simulink model "a2024_V2X_6V_Simulink_model"  (R2023b)
settings: Solver=VariableStepAuto  StartTime=0.0  StopTime=30  MaxStep=1e-2  RelTol=1e-3  AbsTol=1e-3
values from neighbouring files (symbols this model uses):
  b = 1.6    [a2024_v2x_matlab_6veh.m]
  mEgo = 1500    [a2024_v2x_matlab_6veh.m]
  Mode = 1    [a2024_v2x_matlab_6veh.m]    (also in v2x_matlab.m; v2x_matlabV2.m; v2x_matlab_6veh.m; v2x_matlab_R.m)
  pilot = (randi(s,[0 1],pilotsPerSym,1)-0.5)*2    [v2x_matlab.m]
  RxPowerV1 = zeros(sizeEgoWP+2, sizeV1WP+2)    [a2024_v2x_matlab_6veh.m]
  RxPowerV2 = zeros(sizeEgoWP+2, sizeV2WP+2)    [a2024_v2x_matlab_6veh.m]
  RxPowerV3 = zeros(sizeEgoWP+2, sizeV3WP+2)    [a2024_v2x_matlab_6veh.m]
  RxPowerV4 = zeros(sizeEgoWP+2, sizeV4WP+2)    [a2024_v2x_matlab_6veh.m]
  RxPowerV5 = zeros(sizeEgoWP+2, sizeV5WP+2)    [a2024_v2x_matlab_6veh.m]
  RxPowerV6 = zeros(sizeEgoWP+2, sizeV6WP+2)    [a2024_v2x_matlab_6veh.m]
  sampleTime = 0.1    [a2024_v2x_matlab_6veh.m]    (also in v2x_matlab.m; v2x_matlabV2.m; v2x_matlab_6veh.m; v2x_matlab_R.m)
  t_gap = 1.4    [a2024_v2x_matlab_6veh.m]
  waypoints = [egoWP(:,2) egoWP(:,1), zeroforwp]    [a2024_v2x_matlab_6veh.m]    (also in misc.m = data.data.ActorSpecifications(1,1).Waypoints(:,[1,2]); v2x_matlab.m = data.data.ActorSpecifications(1,1).Waypoints(:,[1,2]); v2x_matlabV2.m = [5 -1.6 0; v2x_matlab_R.m = [5 -1.6 0)
  ZeroActors = struct(     'ActorID',0,     'Position', [1000 1000 1000],      'Velocity', [0 0 0],      'Roll', 0,      'Pitch', 0,      'Yaw', 0,      'AngularVelocity', [0 0 0])    [v2x_matlabV2.m]    (also in v2x_matlab_R.m)
undefined symbols (not defined in the file or in its folder): driving, PredictionHorizon, Ts
libraries: commofdm x50, commcnvcod2 x39, simulink x34, commdigbbndam3 x31, commblkintrlv2 x26, commdigbbndpm3 x14, simulink_extras x12, drivingscenarioandsensors x3, mpcadaslib x2, commchan3 x1, vehdynlibdriver x1, commrandsrc3 x1
(part 6 of 6)

== matlab function a2024_V2X_6V_Simulink_model/Calculate PDR/PDR V2/MATLAB Function1 ==
  data: u input; y output; Vehicle_ID input
function y = fcn(u, Vehicle_ID)

y = u(:,Vehicle_ID);

== matlab function a2024_V2X_6V_Simulink_model/Calculate PDR/PDR V2/MATLAB Function2 ==
  settings: sampleTime=sampleTime
  data: Vehicle_ID input; u input; y output
function y = fcn(Vehicle_ID, u)

if isempty(u(:,Vehicle_ID)) 
    y = zeros(1,16);
else
    y = u(:,Vehicle_ID);
end

end

== matlab function a2024_V2X_6V_Simulink_model/Subsystem/MATLAB Function1 ==
  settings: sampleTime=inherited
  data: busActors3Test1 input; Actor output size=18; VehicleID input; VehicleData output Bus: Actors; EgoData input Bus: Actors; counter output; rxPower output; RxPower input
  events: trigger input RISING_EDGE_EVENT
function [Actor, VehicleData, counter, rxPower]  = convBus2IntVector(busActors3Test1, VehicleID, EgoData, RxPower)

% Data extracted from actorss bus

%ActorId = BusActors1Actors.Actors(ActorID).ActorID(1:1);
numActors = int16(busActors3Test1.NumActors);
%time = busActors3Test1.Time;
time = int16(busActors3Test1.Time);

ActorID = VehicleID;

posX = busActors3Test1.Actors(ActorID).Position(1:1);
posY = busActors3Test1.Actors(ActorID).Position(2:2);
posZ = busActors3Test1.Actors(ActorID).Position(3:3);
vPos = [posX posY posZ];

vX = busActors3Test1.Actors(ActorID).Velocity(1:1);
vY = busActors3Test1.Actors(ActorID).Velocity(2:2);
vZ = busActors3Test1.Actors(ActorID).Velocity(3:3);

roll = busActors3Test1.Actors(ActorID).Roll(1:1);
pitch = busActors3Test1.Actors(ActorID).Pitch(1:1);
yaw = busActors3Test1.Actors(ActorID).Yaw(1:1);


angularVelocityX = busActors3Test1.Actors(ActorID).AngularVelocity(1:1);
angularVelocityY = busActors3Test1.Actors(ActorID).AngularVelocity(2:2);
angularVelocityZ = busActors3Test1.Actors(ActorID).AngularVelocity(3:3);

VehicleData = busActors3Test1.Actors(VehicleID);


%% Converting the data

ActorID = int16(ActorID)*10;

posMultip = 10;
posX = int16(round(posMultip*posX));
posY = int16(round(posMultip*posY));
posZ = int16(round(posMultip*posZ));

velMultip = 50;
vX = int16(round(velMultip * vX));
vY = int16(round(velMultip * vY));
vZ = int16(round(velMultip * vZ));

rpyMultip = 50;
roll = int16(round(rpyMultip * roll));
pitch = int16(round(rpyMultip * pitch));
yaw = int16(round(rpyMultip * yaw));

angvelMultip = 50;
angularVelocityX = int16(round(angvelMultip * angularVelocityX));
angularVelocityY = int16(round(angvelMultip * angularVelocityY));
angularVelocityZ = int16(round(angvelMultip * angularVelocityZ));

minusones = ones(3,1);
% Output vector
%zerosVector = zeros(9,1);

intVector = [numActors; time; ActorID; posX; posY; posZ; vX; vY; vZ; roll; pitch; yaw; angularVelocityX; angularVelocityY; angularVelocityZ; minusones];

Actor = intVector;

%% Pathloss (freespace)

% EgoPos = [EgoData.Position(2) EgoData.Position(1) EgoData.Position(3)];
EgoPos = EgoData.Position;
dist = norm(vPos - EgoPos);

fc = 5.9e9;  % Carrier frequency
lambda = (physconst('LightSpeed'))/fc;

PL = fspl(dist, lambda);

Pt_dBm = 33;    % [dBm] Transmission power; maximum permissible transmit power level
sigma = rand(1) + 3.2;  % [3.7 +- 0.5] Variance of the shadowing effect in the wireless communication channel
                        % shadowing follows a log-normal random distribution
X = 2*rand(1)-1;      % random variable following a normal distribution with mean 0 and standard deviation 1
SH = sigma * X;

% h_T = 1;
% h_R = 1;
% dF =  (4*h_T*h_R)/lambda
% lambda1 = 1.61; % Pathloss exponent LOS
% lambda2 = 1.85; % Pathloss exponent NLOS

Pr = Pt_dBm - PL - SH; 

% l1 = 10*lambda1*log(dF)
% l2 = 10*lambda2*log(dist/dF)
% Pr = Prt - l1 - l2 + SH;

P_SEN = -60;

%ZeroActors = int16(zeros(15,1));
% 
counter = 0;
% storedPacket = int16(nan(15,1));
% 
% if Pr > P_SEN
%     Actor = intVector;
%     storedPacket = intVector;
%     counter = 0;
% elseif counter < 10
%     Actor = storedPacket;
%     counter = counter + 1;
% end


%disp(storedPacket)


% persistent prev_value;
% if isempty(prev_value)
%     prev_value = int16(nan(15,1)); % Initialize to a default value
% end
% 
% if Pr > P_SEN
%     Actor = intVector;
%     prev_value = intVector;
%     counter = 0;
% elseif counter < 1
%     Actor = prev_value;
%     counter = counter + 1;
% end


%% SNR
bandwidth = 10e6;
F = 6; % [dB] Noise figure
k = physconst('Boltzmann'); % Boltzmann állandó
T = 300; % [K] Abszolút hőmérséklet

%N0 = 10*log10(bandwidth*k*T/1000)
N0 = -103.8277942;


%N0 = -99;
%SNR = Pr - N0;
egoposition = EgoPos(1,1:2);


distEGO = sqrt(sum((RxPower(3:end, 1:2) - EgoPos(1,1:2)).^2, 2));
distV = sqrt(sum((RxPower(1:2, 3:end)' - vPos(1,1:2)).^2, 2));

[EGOvalue, closestEGO] = min(distEGO);
[Vvalue, closestV] = min(distV);


rxPower = RxPower(closestEGO+2, closestV+2);


%SNR = rxPower - N0;

%% Packet counter
counter = 0;

if (Pr > P_SEN)
    counter = counter + 1;
end

end

== matlab function a2024_V2X_6V_Simulink_model/Calculate PDR/PDR V2/MATLAB Function6 ==
  data: u input; y output Bus: Actors; vehicleID input
function y = fcn(u,vehicleID)

actorsCount = size(u,1);

MinusOneActor = struct(...
    'ActorID',0,...
    'Position', [0 0 0], ...
    'Velocity', [0 0 0], ...
    'Roll', 0, ...
    'Pitch', 0, ...
    'Yaw', 0, ...
    'AngularVelocity', [0 0 0]);

if actorsCount < vehicleID
    y = MinusOneActor;
else
    y = u(:,vehicleID);
end
end

== matlab function a2024_V2X_6V_Simulink_model/Calculate PDR/PDR V3/MATLAB Function ==
  settings: updateMethod=DISCRETE  sampleTime=sampleTime
  data: Tx input; PDR output; Rx input
function PDR = PDR(Tx, Rx)

    
    persistent N S Tx_buffer Rx_buffer

    buffer_size = 20;

    if isempty(N) || isempty(S) || isempty(Tx_buffer) || isempty(Rx_buffer)
        N = 0;
        S = 0;
        Tx_buffer = int16(zeros(buffer_size, length(Tx)));
        Rx_buffer = int16(zeros(buffer_size, length(Rx)));
    end

    Tx_buffer = [Tx_buffer(2:end, :); Tx'];
    Rx_buffer = [Rx_buffer(2:end, :); Rx'];

    if isequal(Tx, Rx) % Check if the entire vectors are the same
        N = N + 1;      % Increment the correct packet count
    end
    S = S + 1;          % Increment the total count
    
    % Calculate the PDR for the last 10 packets
    N_last10 = sum(all(Tx_buffer == Rx_buffer, 2));
    S_last10 = buffer_size;
    R_last10 = (N_last10/S_last10)*100; % Calculate the packet delivery rate [%] for the last 10 packets
    
    R = (N/S)*100;       % Calculate the packet delivery rate [%]
    PDR = [R; N; S; R_last10];
end

== matlab function a2024_V2X_6V_Simulink_model/Calculate PDR/PDR V3/MATLAB Function1 ==
  data: u input; y output; Vehicle_ID input
function y = fcn(u, Vehicle_ID)

y = u(:,Vehicle_ID);

== matlab function a2024_V2X_6V_Simulink_model/Calculate PDR/PDR V3/MATLAB Function2 ==
  settings: sampleTime=sampleTime
  data: Vehicle_ID input; u input; y output
function y = fcn(Vehicle_ID, u)

if isempty(u(:,Vehicle_ID)) 
    y = zeros(1,16);
else
    y = u(:,Vehicle_ID);
end

end

== matlab function a2024_V2X_6V_Simulink_model/Calculate PDR/PDR V3/MATLAB Function6 ==
  data: u input; y output Bus: Actors; vehicleID input
function y = fcn(u,vehicleID)

actorsCount = size(u,1);

MinusOneActor = struct(...
    'ActorID',0,...
    'Position', [0 0 0], ...
    'Velocity', [0 0 0], ...
    'Roll', 0, ...
    'Pitch', 0, ...
    'Yaw', 0, ...
    'AngularVelocity', [0 0 0]);

if actorsCount < vehicleID
    y = MinusOneActor;
else
    y = u(:,vehicleID);
end
end

== matlab function a2024_V2X_6V_Simulink_model/Calculate PDR/PDR V4/MATLAB Function ==
  settings: updateMethod=DISCRETE  sampleTime=sampleTime
  data: Tx input; PDR output; Rx input
function PDR = PDR(Tx, Rx)

    
    persistent N S Tx_buffer Rx_buffer

    buffer_size = 20;

    if isempty(N) || isempty(S) || isempty(Tx_buffer) || isempty(Rx_buffer)
        N = 0;
        S = 0;
        Tx_buffer = int16(zeros(buffer_size, length(Tx)));
        Rx_buffer = int16(zeros(buffer_size, length(Rx)));
    end

    Tx_buffer = [Tx_buffer(2:end, :); Tx'];
    Rx_buffer = [Rx_buffer(2:end, :); Rx'];

    if isequal(Tx, Rx) % Check if the entire vectors are the same
        N = N + 1;      % Increment the correct packet count
    end
    S = S + 1;          % Increment the total count
    
    % Calculate the PDR for the last 10 packets
    N_last10 = sum(all(Tx_buffer == Rx_buffer, 2));
    S_last10 = buffer_size;
    R_last10 = (N_last10/S_last10)*100; % Calculate the packet delivery rate [%] for the last 10 packets
    
    R = (N/S)*100;       % Calculate the packet delivery rate [%]
    PDR = [R; N; S; R_last10];
end

== matlab function a2024_V2X_6V_Simulink_model/Calculate PDR/PDR V4/MATLAB Function1 ==
  data: u input; y output; Vehicle_ID input
function y = fcn(u, Vehicle_ID)

y = u(:,Vehicle_ID);

== matlab function a2024_V2X_6V_Simulink_model/Calculate PDR/PDR V4/MATLAB Function2 ==
  settings: sampleTime=sampleTime
  data: Vehicle_ID input; u input; y output
function y = fcn(Vehicle_ID, u)

if isempty(u(:,Vehicle_ID)) 
    y = zeros(1,16);
else
    y = u(:,Vehicle_ID);
end

end

== matlab function a2024_V2X_6V_Simulink_model/Calculate PDR/PDR V1/MATLAB Function ==
  settings: updateMethod=DISCRETE  sampleTime=sampleTime
  data: Tx input; PDR output; Rx input
function PDR = PDR(Tx, Rx)

    
    persistent N S Tx_buffer Rx_buffer

    buffer_size = 20;

    if isempty(N) || isempty(S) || isempty(Tx_buffer) || isempty(Rx_buffer)
        N = 0;
        S = 0;
        Tx_buffer = int16(zeros(buffer_size, length(Tx)));
        Rx_buffer = int16(zeros(buffer_size, length(Rx)));
    end

    Tx_buffer = [Tx_buffer(2:end, :); Tx'];
    Rx_buffer = [Rx_buffer(2:end, :); Rx'];

    if isequal(Tx, Rx) % Check if the entire vectors are the same
        N = N + 1;      % Increment the correct packet count
    end
    S = S + 1;          % Increment the total count
    
    % Calculate the PDR for the last 10 packets
    N_last10 = sum(all(Tx_buffer == Rx_buffer, 2));
    S_last10 = buffer_size;
    R_last10 = (N_last10/S_last10)*100; % Calculate the packet delivery rate [%] for the last 10 packets
    
    R = (N/S)*100;       % Calculate the packet delivery rate [%]
    PDR = [R; N; S; R_last10];
end

== matlab function a2024_V2X_6V_Simulink_model/Calculate PDR/PDR V1/MATLAB Function2 ==
  settings: sampleTime=sampleTime
  data: Vehicle_ID input; u input; y output
function y = fcn(Vehicle_ID, u)

if isempty(u(:,Vehicle_ID)) 
    y = zeros(1,16);
else
    y = u(:,Vehicle_ID);
end

end

== matlab function a2024_V2X_6V_Simulink_model/Calculate PDR/PDR V1/MATLAB Function6 ==
  data: u input; y output Bus: Actors; vehicleID input
function y = fcn(u,vehicleID)

actorsCount = size(u,1);

MinusOneActor = struct(...
    'ActorID',0,...
    'Position', [0 0 0], ...
    'Velocity', [0 0 0], ...
    'Roll', 0, ...
    'Pitch', 0, ...
    'Yaw', 0, ...
    'AngularVelocity', [0 0 0]);

if actorsCount < vehicleID
    y = MinusOneActor;
else
    y = u(:,vehicleID);
end
end

== matlab function a2024_V2X_6V_Simulink_model/Calculate PDR/PDR V4/MATLAB Function6 ==
  data: u input; y output Bus: Actors; vehicleID input
function y = fcn(u,vehicleID)

actorsCount = size(u,1);

MinusOneActor = struct(...
    'ActorID',0,...
    'Position', [0 0 0], ...
    'Velocity', [0 0 0], ...
    'Roll', 0, ...
    'Pitch', 0, ...
    'Yaw', 0, ...
    'AngularVelocity', [0 0 0]);

if actorsCount < vehicleID
    y = MinusOneActor;
else
    y = u(:,vehicleID);
end
end

== matlab function a2024_V2X_6V_Simulink_model/Calculate PDR/PDR V5/MATLAB Function ==
  settings: updateMethod=DISCRETE  sampleTime=sampleTime
  data: Tx input; PDR output; Rx input
function PDR = PDR(Tx, Rx)

    
    persistent N S Tx_buffer Rx_buffer

    buffer_size = 20;

    if isempty(N) || isempty(S) || isempty(Tx_buffer) || isempty(Rx_buffer)
        N = 0;
        S = 0;
        Tx_buffer = int16(zeros(buffer_size, length(Tx)));
        Rx_buffer = int16(zeros(buffer_size, length(Rx)));
    end

    Tx_buffer = [Tx_buffer(2:end, :); Tx'];
    Rx_buffer = [Rx_buffer(2:end, :); Rx'];

    if isequal(Tx, Rx) % Check if the entire vectors are the same
        N = N + 1;      % Increment the correct packet count
    end
    S = S + 1;          % Increment the total count
    
    % Calculate the PDR for the last 10 packets
    N_last10 = sum(all(Tx_buffer == Rx_buffer, 2));
    S_last10 = buffer_size;
    R_last10 = (N_last10/S_last10)*100; % Calculate the packet delivery rate [%] for the last 10 packets
    
    R = (N/S)*100;       % Calculate the packet delivery rate [%]
    PDR = [R; N; S; R_last10];
end

== matlab function a2024_V2X_6V_Simulink_model/Calculate PDR/PDR V5/MATLAB Function1 ==
  data: u input; y output; Vehicle_ID input
function y = fcn(u, Vehicle_ID)

y = u(:,Vehicle_ID);

== matlab function a2024_V2X_6V_Simulink_model/Subsystem7/MATLAB Function2 ==
  settings: sampleTime=sampleTime
  data: input input; Actors output
function Actors = getRealValues(input) 

modulated = input;

NumActors = modulated(1,:);
Time = modulated(2,:);

ActorID = modulated(3,1)/10;

posMultip = 10;  % 10
posX = (modulated(4,:)/posMultip);
posY = (modulated(5,:)/posMultip);
posZ = (modulated(6,:)/posMultip);

velMultip = 50;  % 50
vX = (modulated(7,:)/velMultip);
vY = (modulated(8,:)/velMultip);
vZ = (modulated(9,:)/velMultip);

rpyMultip = 50;  % 50
Roll = (modulated(10,:)/rpyMultip);
Pitch = (modulated(11,:)/rpyMultip);
Yaw = (modulated(12,:)/rpyMultip);

angvelMultip = 50;  % 50
angularVelocityX = (modulated(13,:)/angvelMultip);
angularVelocityY = (modulated(14,:)/angvelMultip);
angularVelocityZ = (modulated(15,:)/angvelMultip);

% Velocity = [vX vY vZ];
% Position = [posX posY posZ];
% AngularVelocity = [angularVelocityX; angularVelocityY; angularVelocityZ];


%Actors = [NumActors; Time; ActorID; Position; Velocity; Roll; Pitch; Yaw; AngularVelocity];
Actors = [NumActors; Time; ActorID; posX; posY; posZ; vX; vY; vZ; Roll; Pitch; Yaw; angularVelocityX; angularVelocityY; angularVelocityZ];


end

== matlab function a2024_V2X_6V_Simulink_model/Subsystem8/MATLAB Function ==
  settings: updateMethod=DISCRETE  sampleTime=sampleTime
  data: SNR input; modulated input; disrupted_Signal output
function disrupted_Signal = PRO_error(SNR, modulated)

disrupted_Signal = awgn(modulated,SNR, -10);

== matlab function a2024_V2X_6V_Simulink_model/Subsystem8/MATLAB Function1 ==
  settings: sampleTime=inherited
  data: busActors3Test1 input; Actor output size=18; VehicleID input; VehicleData output Bus: Actors; EgoData input Bus: Actors; counter output; rxPower output; RxPower input
  events: trigger input RISING_EDGE_EVENT
function [Actor, VehicleData, counter, rxPower]  = convBus2IntVector(busActors3Test1, VehicleID, EgoData, RxPower)

% Data extracted from actorss bus

%ActorId = BusActors1Actors.Actors(ActorID).ActorID(1:1);
numActors = int16(busActors3Test1.NumActors);
%time = busActors3Test1.Time;
time = int16(busActors3Test1.Time);

ActorID = VehicleID;

posX = busActors3Test1.Actors(ActorID).Position(1:1);
posY = busActors3Test1.Actors(ActorID).Position(2:2);
posZ = busActors3Test1.Actors(ActorID).Position(3:3);
vPos = [posX posY posZ];

vX = busActors3Test1.Actors(ActorID).Velocity(1:1);
vY = busActors3Test1.Actors(ActorID).Velocity(2:2);
vZ = busActors3Test1.Actors(ActorID).Velocity(3:3);

roll = busActors3Test1.Actors(ActorID).Roll(1:1);
pitch = busActors3Test1.Actors(ActorID).Pitch(1:1);
yaw = busActors3Test1.Actors(ActorID).Yaw(1:1);


angularVelocityX = busActors3Test1.Actors(ActorID).AngularVelocity(1:1);
angularVelocityY = busActors3Test1.Actors(ActorID).AngularVelocity(2:2);
angularVelocityZ = busActors3Test1.Actors(ActorID).AngularVelocity(3:3);

VehicleData = busActors3Test1.Actors(VehicleID);


%% Converting the data

ActorID = int16(ActorID)*10;

posMultip = 10;
posX = int16(round(posMultip*posX));
posY = int16(round(posMultip*posY));
posZ = int16(round(posMultip*posZ));

velMultip = 50;
vX = int16(round(velMultip * vX));
vY = int16(round(velMultip * vY));
vZ = int16(round(velMultip * vZ));

rpyMultip = 50;
roll = int16(round(rpyMultip * roll));
pitch = int16(round(rpyMultip * pitch));
yaw = int16(round(rpyMultip * yaw));

angvelMultip = 50;
angularVelocityX = int16(round(angvelMultip * angularVelocityX));
angularVelocityY = int16(round(angvelMultip * angularVelocityY));
angularVelocityZ = int16(round(angvelMultip * angularVelocityZ));

minusones = ones(3,1);
% Output vector
%zerosVector = zeros(9,1);

intVector = [numActors; time; ActorID; posX; posY; posZ; vX; vY; vZ; roll; pitch; yaw; angularVelocityX; angularVelocityY; angularVelocityZ; minusones];

Actor = intVector;

%% Pathloss (freespace)

EgoPos = EgoData.Position;
dist = norm(vPos - EgoPos);

fc = 5.9e9;  % Carrier frequency
lambda = (physconst('LightSpeed'))/fc;

PL = fspl(dist, lambda);

Pt_dBm = 33;    % [dBm] Transmission power; maximum permissible transmit power level
sigma = rand(1) + 3.2;  % [3.7 +- 0.5] Variance of the shadowing effect in the wireless communication channel
                        % shadowing follows a log-normal random distribution
X = 2*rand(1)-1;      % random variable following a normal distribution with mean 0 and standard deviation 1
SH = sigma * X;

% h_T = 1;
% h_R = 1;
% dF =  (4*h_T*h_R)/lambda
% lambda1 = 1.61; % Pathloss exponent LOS
% lambda2 = 1.85; % Pathloss exponent NLOS

Pr = Pt_dBm - PL - SH; 

% l1 = 10*lambda1*log(dF)
% l2 = 10*lambda2*log(dist/dF)
% Pr = Prt - l1 - l2 + SH;

P_SEN = -60;

%ZeroActors = int16(zeros(15,1));
% 
counter = 0;
% storedPacket = int16(nan(15,1));
% 
% if Pr > P_SEN
%     Actor = intVector;
%     storedPacket = intVector;
%     counter = 0;
% elseif counter < 10
%     Actor = storedPacket;
%     counter = counter + 1;
% end


%disp(storedPacket)


% persistent prev_value;
% if isempty(prev_value)
%     prev_value = int16(nan(15,1)); % Initialize to a default value
% end
% 
% if Pr > P_SEN
%     Actor = intVector;
%     prev_value = intVector;
%     counter = 0;
% elseif counter < 1
%     Actor = prev_value;
%     counter = counter + 1;
% end


%% SNR
bandwidth = 10e6;
F = 6; % [dB] Noise figure
k = physconst('Boltzmann'); % Boltzmann állandó
T = 300; % [K] Abszolút hőmérséklet

%N0 = 10*log10(bandwidth*k*T/1000)
N0 = -103.8277942;


%N0 = -99;
%SNR = Pr - N0;
egoposition = EgoPos(1,1:2);


distEGO = sqrt(sum((RxPower(3:end, 1:2) - EgoPos(1,1:2)).^2, 2));
distV = sqrt(sum((RxPower(1:2, 3:end)' - vPos(1,1:2)).^2, 2));

[EGOvalue, closestEGO] = min(distEGO);
[Vvalue, closestV] = min(distV);


rxPower = RxPower(closestEGO+2, closestV+2);


%SNR = rxPower - N0;

%% Packet counter
counter = 0;

if (Pr > P_SEN)
    counter = counter + 1;
end

end

== matlab function a2024_V2X_6V_Simulink_model/Subsystem3/MATLAB Function2 ==
  settings: sampleTime=sampleTime
  data: input input; Actors output
function Actors = getRealValues(input) 

modulated = input(1:15);

NumActors = modulated(1,:);
Time = modulated(2,:);

ActorID = ((modulated(3,1))/10);

posMultip = 10;  % 10
posX = (modulated(4,:)/posMultip);
posY = (modulated(5,:)/posMultip);
posZ = (modulated(6,:)/posMultip);

velMultip = 50;  % 50
vX = (modulated(7,:)/velMultip);
vY = (modulated(8,:)/velMultip);
vZ = (modulated(9,:)/velMultip);

rpyMultip = 50;  % 50
Roll = (modulated(10,:)/rpyMultip);
Pitch = (modulated(11,:)/rpyMultip);
Yaw = (modulated(12,:)/rpyMultip);

angvelMultip = 50;  % 50
angularVelocityX = (modulated(13,:)/angvelMultip);
angularVelocityY = (modulated(14,:)/angvelMultip);
angularVelocityZ = (modulated(15,:)/angvelMultip);

% Velocity = [vX vY vZ];
% Position = [posX posY posZ];
% AngularVelocity = [angularVelocityX; angularVelocityY; angularVelocityZ];


%Actors = [NumActors; Time; ActorID; Position; Velocity; Roll; Pitch; Yaw; AngularVelocity];
Actors = [NumActors; Time; ActorID; posX; posY; posZ; vX; vY; vZ; Roll; Pitch; Yaw; angularVelocityX; angularVelocityY; angularVelocityZ];


end

== matlab function a2024_V2X_6V_Simulink_model/Subsystem8/MATLAB Function2 ==
  settings: sampleTime=sampleTime
  data: input input; Actors output
function Actors = getRealValues(input) 

modulated = input;

NumActors = modulated(1,:);
Time = modulated(2,:);

ActorID = modulated(3,1)/10;

posMultip = 10;  % 10
posX = (modulated(4,:)/posMultip);
posY = (modulated(5,:)/posMultip);
posZ = (modulated(6,:)/posMultip);

velMultip = 50;  % 50
vX = (modulated(7,:)/velMultip);
vY = (modulated(8,:)/velMultip);
vZ = (modulated(9,:)/velMultip);

rpyMultip = 50;  % 50
Roll = (modulated(10,:)/rpyMultip);
Pitch = (modulated(11,:)/rpyMultip);
Yaw = (modulated(12,:)/rpyMultip);

angvelMultip = 50;  % 50
angularVelocityX = (modulated(13,:)/angvelMultip);
angularVelocityY = (modulated(14,:)/angvelMultip);
angularVelocityZ = (modulated(15,:)/angvelMultip);

% Velocity = [vX vY vZ];
% Position = [posX posY posZ];
% AngularVelocity = [angularVelocityX; angularVelocityY; angularVelocityZ];


%Actors = [NumActors; Time; ActorID; Position; Velocity; Roll; Pitch; Yaw; AngularVelocity];
Actors = [NumActors; Time; ActorID; posX; posY; posZ; vX; vY; vZ; Roll; Pitch; Yaw; angularVelocityX; angularVelocityY; angularVelocityZ];


end

== matlab function a2024_V2X_6V_Simulink_model/Calculate PDR/PDR V5/MATLAB Function2 ==
  settings: sampleTime=sampleTime
  data: Vehicle_ID input; u input; y output
function y = fcn(Vehicle_ID, u)

if isempty(u(:,Vehicle_ID)) 
    y = zeros(1,16);
else
    y = u(:,Vehicle_ID);
end

end

== matlab function a2024_V2X_6V_Simulink_model/Calculate PDR/PDR V5/MATLAB Function6 ==
  data: u input; y output Bus: Actors; vehicleID input
function y = fcn(u,vehicleID)

actorsCount = size(u,1);

MinusOneActor = struct(...
    'ActorID',0,...
    'Position', [0 0 0], ...
    'Velocity', [0 0 0], ...
    'Roll', 0, ...
    'Pitch', 0, ...
    'Yaw', 0, ...
    'AngularVelocity', [0 0 0]);

if actorsCount < vehicleID
    y = MinusOneActor;
else
    y = u(:,vehicleID);
end
end

== matlab function a2024_V2X_6V_Simulink_model/Subsystem9/MATLAB Function2 ==
  settings: sampleTime=sampleTime
  data: input input; Actors output
function Actors = getRealValues(input) 

modulated = input(1:15);

NumActors = modulated(1,:);
Time = modulated(2,:);

ActorID = ((modulated(3,1))/10);

posMultip = 10;  % 10
posX = (modulated(4,:)/posMultip);
posY = (modulated(5,:)/posMultip);
posZ = (modulated(6,:)/posMultip);

velMultip = 50;  % 50
vX = (modulated(7,:)/velMultip);
vY = (modulated(8,:)/velMultip);
vZ = (modulated(9,:)/velMultip);

rpyMultip = 50;  % 50
Roll = (modulated(10,:)/rpyMultip);
Pitch = (modulated(11,:)/rpyMultip);
Yaw = (modulated(12,:)/rpyMultip);

angvelMultip = 50;  % 50
angularVelocityX = (modulated(13,:)/angvelMultip);
angularVelocityY = (modulated(14,:)/angvelMultip);
angularVelocityZ = (modulated(15,:)/angvelMultip);

% Velocity = [vX vY vZ];
% Position = [posX posY posZ];
% AngularVelocity = [angularVelocityX; angularVelocityY; angularVelocityZ];


%Actors = [NumActors; Time; ActorID; Position; Velocity; Roll; Pitch; Yaw; AngularVelocity];
Actors = [NumActors; Time; ActorID; posX; posY; posZ; vX; vY; vZ; Roll; Pitch; Yaw; angularVelocityX; angularVelocityY; angularVelocityZ];


end

== matlab function a2024_V2X_6V_Simulink_model/Calculate PDR/PDR V6/MATLAB Function ==
  settings: updateMethod=DISCRETE  sampleTime=sampleTime
  data: Tx input; PDR output; Rx input
function PDR = PDR(Tx, Rx)

    
    persistent N S Tx_buffer Rx_buffer

    buffer_size = 20;

    if isempty(N) || isempty(S) || isempty(Tx_buffer) || isempty(Rx_buffer)
        N = 0;
        S = 0;
        Tx_buffer = int16(zeros(buffer_size, length(Tx)));
        Rx_buffer = int16(zeros(buffer_size, length(Rx)));
    end

    Tx_buffer = [Tx_buffer(2:end, :); Tx'];
    Rx_buffer = [Rx_buffer(2:end, :); Rx'];

    if isequal(Tx, Rx) % Check if the entire vectors are the same
        N = N + 1;      % Increment the correct packet count
    end
    S = S + 1;          % Increment the total count
    
    % Calculate the PDR for the last 10 packets
    N_last10 = sum(all(Tx_buffer == Rx_buffer, 2));
    S_last10 = buffer_size;
    R_last10 = (N_last10/S_last10)*100; % Calculate the packet delivery rate [%] for the last 10 packets
    
    R = (N/S)*100;       % Calculate the packet delivery rate [%]
    PDR = [R; N; S; R_last10];
end

== matlab function a2024_V2X_6V_Simulink_model/Calculate PDR/PDR V6/MATLAB Function1 ==
  data: u input; y output; Vehicle_ID input
function y = fcn(u, Vehicle_ID)

y = u(:,Vehicle_ID);

== matlab function a2024_V2X_6V_Simulink_model/Calculate PDR/PDR V6/MATLAB Function2 ==
  settings: sampleTime=sampleTime
  data: Vehicle_ID input; u input; y output
function y = fcn(Vehicle_ID, u)

if isempty(u(:,Vehicle_ID)) 
    y = zeros(1,16);
else
    y = u(:,Vehicle_ID);
end

end

== matlab function a2024_V2X_6V_Simulink_model/Calculate PDR/PDR V6/MATLAB Function6 ==
  data: u input; y output Bus: Actors; vehicleID input
function y = fcn(u,vehicleID)

actorsCount = size(u,1);

MinusOneActor = struct(...
    'ActorID',0,...
    'Position', [0 0 0], ...
    'Velocity', [0 0 0], ...
    'Roll', 0, ...
    'Pitch', 0, ...
    'Yaw', 0, ...
    'AngularVelocity', [0 0 0]);

if actorsCount < vehicleID
    y = MinusOneActor;
else
    y = u(:,vehicleID);
end
end

== matlab function a2024_V2X_6V_Simulink_model/Subsystem10/MATLAB Function2 ==
  settings: sampleTime=sampleTime
  data: input input; Actors output
function Actors = getRealValues(input) 

modulated = input(1:15);

NumActors = modulated(1,:);
Time = modulated(2,:);

ActorID = ((modulated(3,1))/10);

posMultip = 10;  % 10
posX = (modulated(4,:)/posMultip);
posY = (modulated(5,:)/posMultip);
posZ = (modulated(6,:)/posMultip);

velMultip = 50;  % 50
vX = (modulated(7,:)/velMultip);
vY = (modulated(8,:)/velMultip);
vZ = (modulated(9,:)/velMultip);

rpyMultip = 50;  % 50
Roll = (modulated(10,:)/rpyMultip);
Pitch = (modulated(11,:)/rpyMultip);
Yaw = (modulated(12,:)/rpyMultip);

angvelMultip = 50;  % 50
angularVelocityX = (modulated(13,:)/angvelMultip);
angularVelocityY = (modulated(14,:)/angvelMultip);
angularVelocityZ = (modulated(15,:)/angvelMultip);

% Velocity = [vX vY vZ];
% Position = [posX posY posZ];
% AngularVelocity = [angularVelocityX; angularVelocityY; angularVelocityZ];


%Actors = [NumActors; Time; ActorID; Position; Velocity; Roll; Pitch; Yaw; AngularVelocity];
Actors = [NumActors; Time; ActorID; posX; posY; posZ; vX; vY; vZ; Roll; Pitch; Yaw; angularVelocityX; angularVelocityY; angularVelocityZ];


end

== matlab function a2024_V2X_6V_Simulink_model/Subsystem4/MATLAB Function ==
  settings: updateMethod=DISCRETE  sampleTime=sampleTime
  data: SNR input; modulated input; disrupted_Signal output
function disrupted_Signal = PRO_error(SNR, modulated)

disrupted_Signal = awgn(modulated,SNR, -10);

== matlab function a2024_V2X_6V_Simulink_model/Subsystem11/MATLAB Function2 ==
  settings: sampleTime=sampleTime
  data: input input; Actors output
function Actors = getRealValues(input) 

modulated = input(1:15);

NumActors = modulated(1,:);
Time = modulated(2,:);

ActorID = ((modulated(3,1))/10);

posMultip = 10;  % 10
posX = (modulated(4,:)/posMultip);
posY = (modulated(5,:)/posMultip);
posZ = (modulated(6,:)/posMultip);

velMultip = 50;  % 50
vX = (modulated(7,:)/velMultip);
vY = (modulated(8,:)/velMultip);
vZ = (modulated(9,:)/velMultip);

rpyMultip = 50;  % 50
Roll = (modulated(10,:)/rpyMultip);
Pitch = (modulated(11,:)/rpyMultip);
Yaw = (modulated(12,:)/rpyMultip);

angvelMultip = 50;  % 50
angularVelocityX = (modulated(13,:)/angvelMultip);
angularVelocityY = (modulated(14,:)/angvelMultip);
angularVelocityZ = (modulated(15,:)/angvelMultip);

% Velocity = [vX vY vZ];
% Position = [posX posY posZ];
% AngularVelocity = [angularVelocityX; angularVelocityY; angularVelocityZ];


%Actors = [NumActors; Time; ActorID; Position; Velocity; Roll; Pitch; Yaw; AngularVelocity];
Actors = [NumActors; Time; ActorID; posX; posY; posZ; vX; vY; vZ; Roll; Pitch; Yaw; angularVelocityX; angularVelocityY; angularVelocityZ];


end

== matlab function a2024_V2X_6V_Simulink_model/Subsystem12/MATLAB Function2 ==
  settings: sampleTime=sampleTime
  data: input input; Actors output
function Actors = getRealValues(input) 

modulated = input(1:15);

NumActors = modulated(1,:);
Time = modulated(2,:);

ActorID = ((modulated(3,1))/10);

posMultip = 10;  % 10
posX = (modulated(4,:)/posMultip);
posY = (modulated(5,:)/posMultip);
posZ = (modulated(6,:)/posMultip);

velMultip = 50;  % 50
vX = (modulated(7,:)/velMultip);
vY = (modulated(8,:)/velMultip);
vZ = (modulated(9,:)/velMultip);

rpyMultip = 50;  % 50
Roll = (modulated(10,:)/rpyMultip);
Pitch = (modulated(11,:)/rpyMultip);
Yaw = (modulated(12,:)/rpyMultip);

angvelMultip = 50;  % 50
angularVelocityX = (modulated(13,:)/angvelMultip);
angularVelocityY = (modulated(14,:)/angvelMultip);
angularVelocityZ = (modulated(15,:)/angvelMultip);

% Velocity = [vX vY vZ];
% Position = [posX posY posZ];
% AngularVelocity = [angularVelocityX; angularVelocityY; angularVelocityZ];


%Actors = [NumActors; Time; ActorID; Position; Velocity; Roll; Pitch; Yaw; AngularVelocity];
Actors = [NumActors; Time; ActorID; posX; posY; posZ; vX; vY; vZ; Roll; Pitch; Yaw; angularVelocityX; angularVelocityY; angularVelocityZ];


end

== matlab function a2024_V2X_6V_Simulink_model/Subsystem13/MATLAB Function2 ==
  settings: sampleTime=sampleTime
  data: input input; Actors output
function Actors = getRealValues(input) 

modulated = input(1:15);

NumActors = modulated(1,:);
Time = modulated(2,:);

ActorID = ((modulated(3,1))/10);

posMultip = 10;  % 10
posX = (modulated(4,:)/posMultip);
posY = (modulated(5,:)/posMultip);
posZ = (modulated(6,:)/posMultip);

velMultip = 50;  % 50
vX = (modulated(7,:)/velMultip);
vY = (modulated(8,:)/velMultip);
vZ = (modulated(9,:)/velMultip);

rpyMultip = 50;  % 50
Roll = (modulated(10,:)/rpyMultip);
Pitch = (modulated(11,:)/rpyMultip);
Yaw = (modulated(12,:)/rpyMultip);

angvelMultip = 50;  % 50
angularVelocityX = (modulated(13,:)/angvelMultip);
angularVelocityY = (modulated(14,:)/angvelMultip);
angularVelocityZ = (modulated(15,:)/angvelMultip);

% Velocity = [vX vY vZ];
% Position = [posX posY posZ];
% AngularVelocity = [angularVelocityX; angularVelocityY; angularVelocityZ];


%Actors = [NumActors; Time; ActorID; Position; Velocity; Roll; Pitch; Yaw; AngularVelocity];
Actors = [NumActors; Time; ActorID; posX; posY; posZ; vX; vY; vZ; Roll; Pitch; Yaw; angularVelocityX; angularVelocityY; angularVelocityZ];


end

== matlab function a2024_V2X_6V_Simulink_model/Subsystem14/MATLAB Function2 ==
  settings: sampleTime=sampleTime
  data: input input; Actors output
function Actors = getRealValues(input) 

modulated = input(1:15);

NumActors = modulated(1,:);
Time = modulated(2,:);

ActorID = ((modulated(3,1))/10);

posMultip = 10;  % 10
posX = (modulated(4,:)/posMultip);
posY = (modulated(5,:)/posMultip);
posZ = (modulated(6,:)/posMultip);

velMultip = 50;  % 50
vX = (modulated(7,:)/velMultip);
vY = (modulated(8,:)/velMultip);
vZ = (modulated(9,:)/velMultip);

rpyMultip = 50;  % 50
Roll = (modulated(10,:)/rpyMultip);
Pitch = (modulated(11,:)/rpyMultip);
Yaw = (modulated(12,:)/rpyMultip);

angvelMultip = 50;  % 50
angularVelocityX = (modulated(13,:)/angvelMultip);
angularVelocityY = (modulated(14,:)/angvelMultip);
angularVelocityZ = (modulated(15,:)/angvelMultip);

% Velocity = [vX vY vZ];
% Position = [posX posY posZ];
% AngularVelocity = [angularVelocityX; angularVelocityY; angularVelocityZ];


%Actors = [NumActors; Time; ActorID; Position; Velocity; Roll; Pitch; Yaw; AngularVelocity];
Actors = [NumActors; Time; ActorID; posX; posY; posZ; vX; vY; vZ; Roll; Pitch; Yaw; angularVelocityX; angularVelocityY; angularVelocityZ];


end

== matlab function a2024_V2X_6V_Simulink_model/MATLAB Function ==
  data: V1Actor input; relDist output; EgoActor input; relVel output; EgoPos output
function [relDist, relVel, EgoPos] = fcn(V1Actor, EgoActor)


EgoPos = double(EgoActor.Position);
EgoVel = double(EgoActor.Velocity);

V1Pos = double(V1Actor(4:6,1))';
V1Vel = double(V1Actor(7:9,1))';

if isequal(V1Pos, zeros(1,3))
    V1Pos = [170 3 0];
    V1Vel = [0, -7, 0];
end


%EgoPosNorm = norm(EgoPos);
%V1PosNorm = norm(V1Pos);

%possquared = (EgoPos(1) - V1Pos(1))^2 + (EgoPos(2) - V1Pos(2))^2;

%EgoVelNorm = norm(EgoVel);
%V1VelNorm = norm(V1Vel);

%velsquared = (EgoVel(1) - V1Vel(1))^2 + (EgoVel(2) - V1Vel(2))^2;

%relDist = sqrt(possquared);
relDist = V1Pos - EgoPos;
%relVel = sqrt(velsquared)
relVel = V1Vel - EgoVel;

% relDist = sqrt((((EgoPos(1) - V1Pos(1)).^2)+((EgoPos(2) - V1Pos(2))).^2), 2);
% relVel = sqrt((((EgoVel(1) - V1Vel(1)).^2)+((EgoVel(2) - V1Vel(2))).^2), 2);

% relDist = norm(V1Pos - EgoPos);
% relVel = norm(V1Vel - EgoVel);

== matlab function a2024_V2X_6V_Simulink_model/Vehicle 3/MATLAB Function2 ==
  data: busActors3Test1 input; intVector output int16 size=15; VehicleID input
  events: trigger input RISING_EDGE_EVENT
function intVector = convBus2IntVector(busActors3Test1, VehicleID)

% Data extracted from actorss bus

%ActorId = BusActors1Actors.Actors(ActorID).ActorID(1:1);
numActors = busActors3Test1.NumActors;
time = busActors3Test1.Time;

ActorID = VehicleID;

posX = busActors3Test1.Actors(ActorID).Position(1:1);
posY = busActors3Test1.Actors(ActorID).Position(2:2);
posZ = busActors3Test1.Actors(ActorID).Position(3:3);

vX = busActors3Test1.Actors(ActorID).Velocity(1:1);
vY = busActors3Test1.Actors(ActorID).Velocity(2:2);
vZ = busActors3Test1.Actors(ActorID).Velocity(3:3);

roll = busActors3Test1.Actors(ActorID).Roll(1:1);
pitch = busActors3Test1.Actors(ActorID).Pitch(1:1);
yaw = busActors3Test1.Actors(ActorID).Yaw(1:1);


angularVelocityX = busActors3Test1.Actors(ActorID).AngularVelocity(1:1);
angularVelocityY = busActors3Test1.Actors(ActorID).AngularVelocity(2:2);
angularVelocityZ = busActors3Test1.Actors(ActorID).AngularVelocity(3:3);


% Converting the data

ActorID = int16(ActorID);

posMultip = 10;
posX = int16(round(posMultip*posX));
posY = int16(round(posMultip*posY));
posZ = int16(round(posMultip*posZ));

velMultip = 50;
vX = int16(round(velMultip * vX));
vY = int16(round(velMultip * vY));
vZ = int16(round(velMultip * vZ));

rpyMultip = 50;
roll = int16(round(rpyMultip * roll));
pitch = int16(round(rpyMultip * pitch));
yaw = int16(round(rpyMultip * yaw));

angvelMultip = 50;
angularVelocityX = int16(round(angvelMultip * angularVelocityX));
angularVelocityY = int16(round(angvelMultip * angularVelocityY));
angularVelocityZ = int16(round(angvelMultip * angularVelocityZ));


% Output vector
%zerosVector = zeros(9,1);

intVector = [numActors; time; ActorID; posX; posY; posZ; vX; vY; vZ; roll; pitch; yaw; angularVelocityX; angularVelocityY; angularVelocityZ];
end

== matlab function a2024_V2X_6V_Simulink_model/Subsystem1/MATLAB Function1 ==
  data: busActors3Test1 input; Actor output int16 size=15; VehicleID input; VehicleData output Bus: Actors; EgoData input Bus: Actors; counter output
  events: trigger input RISING_EDGE_EVENT
function [Actor, VehicleData, counter]  = convBus2IntVector(busActors3Test1, VehicleID, EgoData)

% Data extracted from actorss bus

%ActorId = BusActors1Actors.Actors(ActorID).ActorID(1:1);
numActors = busActors3Test1.NumActors;
%time = busActors3Test1.Time;
time = busActors3Test1.Time;

ActorID = VehicleID;

posX = busActors3Test1.Actors(ActorID).Position(1:1);
posY = busActors3Test1.Actors(ActorID).Position(2:2);
posZ = busActors3Test1.Actors(ActorID).Position(3:3);
vPos = [posX posY posZ];

vX = busActors3Test1.Actors(ActorID).Velocity(1:1);
vY = busActors3Test1.Actors(ActorID).Velocity(2:2);
vZ = busActors3Test1.Actors(ActorID).Velocity(3:3);

roll = busActors3Test1.Actors(ActorID).Roll(1:1);
pitch = busActors3Test1.Actors(ActorID).Pitch(1:1);
yaw = busActors3Test1.Actors(ActorID).Yaw(1:1);


angularVelocityX = busActors3Test1.Actors(ActorID).AngularVelocity(1:1);
angularVelocityY = busActors3Test1.Actors(ActorID).AngularVelocity(2:2);
angularVelocityZ = busActors3Test1.Actors(ActorID).AngularVelocity(3:3);

VehicleData = busActors3Test1.Actors(ActorID);


%% Converting the data

ActorID = int16(ActorID);

posMultip = 10;
posX = int16(round(posMultip*posX));
posY = int16(round(posMultip*posY));
posZ = int16(round(posMultip*posZ));

velMultip = 50;
vX = int16(round(velMultip * vX));
vY = int16(round(velMultip * vY));
vZ = int16(round(velMultip * vZ));

rpyMultip = 50;
roll = int16(round(rpyMultip * roll));
pitch = int16(round(rpyMultip * pitch));
yaw = int16(round(rpyMultip * yaw));

angvelMultip = 50;
angularVelocityX = int16(round(angvelMultip * angularVelocityX));
angularVelocityY = int16(round(angvelMultip * angularVelocityY));
angularVelocityZ = int16(round(angvelMultip * angularVelocityZ));


% Output vector
%zerosVector = zeros(9,1);

intVector = [numActors; time; ActorID; posX; posY; posZ; vX; vY; vZ; roll; pitch; yaw; angularVelocityX; angularVelocityY; angularVelocityZ];



%% Pathloss (freespace)

EgoPos = EgoData.Position;
dist = norm(vPos - EgoPos);

fc = 5.9*10^9;  % Carrier frequency
lambda = physconst('LightSpeed')/fc;

PL = fspl(dist, lambda);

Pt_dBm = 33;    % [dBm] Transmission power; maximum permissible transmit power level
sigma = rand(1) + 3.2;  % [3.7 +- 0.5] Variance of the shadowing effect in the wireless communication channel
                        % shadowing follows a log-normal random distribution
X = randn(1);       % random variable following a normal distribution with mean 0 and standard deviation 1
SH = sigma * X;

Pr = Pt_dBm - PL - SH;

P_SEN = -60;

ZeroActors = int16(zeros(15,1));

persistent prev_value;
if isempty(prev_value)
    prev_value = ZeroActors; % Initialize to a default value
end

if Pr > P_SEN
    Actor = intVector;
    prev_value = intVector;
else
    Actor = prev_value;
end


%% Packet counter
counter = 0;

if (Pr > P_SEN)
    counter = counter + 1;
end


end

== matlab function a2024_V2X_6V_Simulink_model/MATLAB Function2 ==
  data: Ego input; EgoActor output; V1 input; V1Actor output
function [EgoActor, V1Actor] = ENU_to_NED(Ego, V1)

T = [cos(nu) -sin(nu) 0 a;
    cos(alpha)*sin(nu) cos(alpha)*cos(nu) -sin(alpha) -d*sin(alpha);
    sin(alpha)*sin(nu) sin(alpha)*cos(nu) cos(alpha) d*cos(alpha);
    0 0 0 1];

== matlab function a2024_V2X_6V_Simulink_model/Subsystem4/MATLAB Function1 ==
  settings: sampleTime=inherited
  data: busActors3Test1 input; Actor output size=18; VehicleID input; VehicleData output Bus: Actors; EgoData input Bus: Actors; counter output; rxPower output; RxPower input
  events: trigger input RISING_EDGE_EVENT
function [Actor, VehicleData, counter, rxPower]  = convBus2IntVector(busActors3Test1, VehicleID, EgoData, RxPower)

% Data extracted from actorss bus

%ActorId = BusActors1Actors.Actors(ActorID).ActorID(1:1);
numActors = int16(busActors3Test1.NumActors);
%time = busActors3Test1.Time;
time = int16(busActors3Test1.Time);

ActorID = VehicleID;

posX = busActors3Test1.Actors(ActorID).Position(1:1);
posY = busActors3Test1.Actors(ActorID).Position(2:2);
posZ = busActors3Test1.Actors(ActorID).Position(3:3);
vPos = [posX posY posZ];

vX = busActors3Test1.Actors(ActorID).Velocity(1:1);
vY = busActors3Test1.Actors(ActorID).Velocity(2:2);
vZ = busActors3Test1.Actors(ActorID).Velocity(3:3);

roll = busActors3Test1.Actors(ActorID).Roll(1:1);
pitch = busActors3Test1.Actors(ActorID).Pitch(1:1);
yaw = busActors3Test1.Actors(ActorID).Yaw(1:1);


angularVelocityX = busActors3Test1.Actors(ActorID).AngularVelocity(1:1);
angularVelocityY = busActors3Test1.Actors(ActorID).AngularVelocity(2:2);
angularVelocityZ = busActors3Test1.Actors(ActorID).AngularVelocity(3:3);

VehicleData = busActors3Test1.Actors(VehicleID);


%% Converting the data

ActorID = int16(ActorID)*10;

posMultip = 10;
posX = int16(round(posMultip*posX));
posY = int16(round(posMultip*posY));
posZ = int16(round(posMultip*posZ));

velMultip = 50;
vX = int16(round(velMultip * vX));
vY = int16(round(velMultip * vY));
vZ = int16(round(velMultip * vZ));

rpyMultip = 50;
roll = int16(round(rpyMultip * roll));
pitch = int16(round(rpyMultip * pitch));
yaw = int16(round(rpyMultip * yaw));

angvelMultip = 50;
angularVelocityX = int16(round(angvelMultip * angularVelocityX));
angularVelocityY = int16(round(angvelMultip * angularVelocityY));
angularVelocityZ = int16(round(angvelMultip * angularVelocityZ));

minusones = ones(3,1);
% Output vector
%zerosVector = zeros(9,1);

intVector = [numActors; time; ActorID; posX; posY; posZ; vX; vY; vZ; roll; pitch; yaw; angularVelocityX; angularVelocityY; angularVelocityZ; minusones];

Actor = intVector;

%% Pathloss (freespace)

EgoPos = EgoData.Position;
dist = norm(vPos - EgoPos);

fc = 5.9e9;  % Carrier frequency
lambda = (physconst('LightSpeed'))/fc;

PL = fspl(dist, lambda);

Pt_dBm = 33;    % [dBm] Transmission power; maximum permissible transmit power level
sigma = rand(1) + 3.2;  % [3.7 +- 0.5] Variance of the shadowing effect in the wireless communication channel
                        % shadowing follows a log-normal random distribution
X = 2*rand(1)-1;      % random variable following a normal distribution with mean 0 and standard deviation 1
SH = sigma * X;

% h_T = 1;
% h_R = 1;
% dF =  (4*h_T*h_R)/lambda
% lambda1 = 1.61; % Pathloss exponent LOS
% lambda2 = 1.85; % Pathloss exponent NLOS

Pr = Pt_dBm - PL - SH; 

% l1 = 10*lambda1*log(dF)
% l2 = 10*lambda2*log(dist/dF)
% Pr = Prt - l1 - l2 + SH;

P_SEN = -60;

%ZeroActors = int16(zeros(15,1));
% 
counter = 0;
% storedPacket = int16(nan(15,1));
% 
% if Pr > P_SEN
%     Actor = intVector;
%     storedPacket = intVector;
%     counter = 0;
% elseif counter < 10
%     Actor = storedPacket;
%     counter = counter + 1;
% end


%disp(storedPacket)


% persistent prev_value;
% if isempty(prev_value)
%     prev_value = int16(nan(15,1)); % Initialize to a default value
% end
% 
% if Pr > P_SEN
%     Actor = intVector;
%     prev_value = intVector;
%     counter = 0;
% elseif counter < 1
%     Actor = prev_value;
%     counter = counter + 1;
% end


%% SNR
bandwidth = 10e6;
F = 6; % [dB] Noise figure
k = physconst('Boltzmann'); % Boltzmann állandó
T = 300; % [K] Abszolút hőmérséklet

%N0 = 10*log10(bandwidth*k*T/1000)
N0 = -103.8277942;


%N0 = -99;
%SNR = Pr - N0;
egoposition = EgoPos(1,1:2);


distEGO = sqrt(sum((RxPower(3:end, 1:2) - EgoPos(1,1:2)).^2, 2));
distV = sqrt(sum((RxPower(1:2, 3:end)' - vPos(1,1:2)).^2, 2));

[EGOvalue, closestEGO] = min(distEGO);
[Vvalue, closestV] = min(distV);

rxPower = RxPower(closestEGO+2, closestV+2);


%SNR = rxPower - N0;

%% Packet counter
counter = 0;

if (Pr > P_SEN)
    counter = counter + 1;
end

end
